simulink model "DPWM_test"  (R2023b)
settings: Solver=VariableStepAuto  StartTime=0.0  StopTime=0.5  MaxStep=0.0001  RelTol=1e-3
libraries: spsMosfetLib x6, spsDCVoltageSourceLib x1, spsGroundLib x1, spsTriangleGeneratorLib x1, spsThreePhaseSeriesRLCBranchLib x1, spsThreePhaseVIMeasurementLib x1, spspowerguiLib x1
settings Model: Creator=oscar  LastModifiedBy=oscar

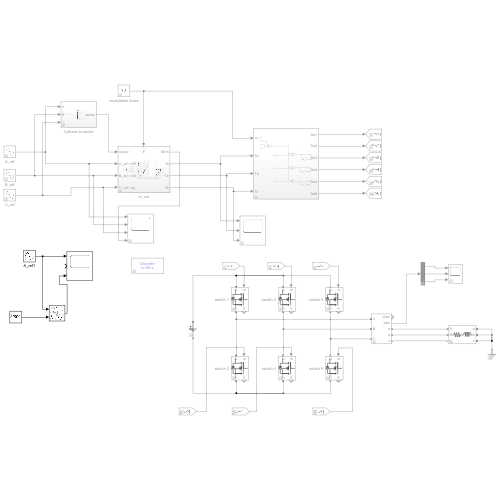
[thumbnail: Simulink's stored preview of the top-level diagram]
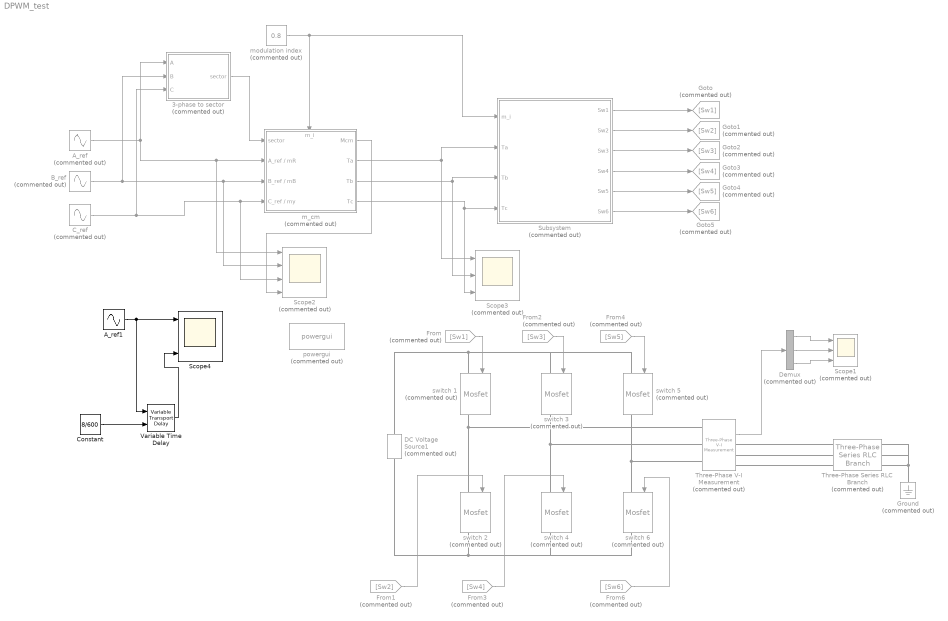
== system DPWM_test ==
  3-phase to sector : Subsystem  Commented=on
  A_ref : Sin  Commented=on  Frequency=2*pi*50  SampleTime=0
  A_ref1 : Sin  Frequency=2*pi*50  SampleTime=0
  B_ref : Sin  Commented=on  Frequency=2*pi*50  Phase=2*pi/3  SampleTime=0
  C_ref : Sin  Commented=on  Frequency=2*pi*50  Phase=4*pi/3  SampleTime=0
  Constant : Constant  Value=8/600
  DC Voltage Source1 : spsDCVoltageSourceLib/DC Voltage Source  Commented=on  Amplitude=100  Measurements=None
  Demux : Demux  Commented=on  Outputs=3
  From : From  Commented=on  GotoTag=Sw1
  From1 : From  Commented=on  GotoTag=Sw2
  From2 : From  Commented=on  GotoTag=Sw3
  From3 : From  Commented=on  GotoTag=Sw4
  From4 : From  Commented=on  GotoTag=Sw5
  From6 : From  Commented=on  GotoTag=Sw6
  Goto : Goto  Commented=on  GotoTag=Sw1
  Goto1 : Goto  Commented=on  GotoTag=Sw2
  Goto2 : Goto  Commented=on  GotoTag=Sw3
  Goto3 : Goto  Commented=on  GotoTag=Sw4
  Goto4 : Goto  Commented=on  GotoTag=Sw5
  Goto5 : Goto  Commented=on  GotoTag=Sw6
  Ground : spsGroundLib/Ground  Commented=on  LConnTagsString=a
  Scope1 : Scope  Commented=on  NumInputPorts=3
  Scope2 : Scope  Commented=on  NumInputPorts=4
  Scope3 : Scope  Commented=on  NumInputPorts=3
  Scope4 : Scope  NumInputPorts=3
  Subsystem : Subsystem  Commented=on
  Three-Phase Series RLC Branch : spsThreePhaseSeriesRLCBranchLib/Three-Phase Series RLC Branch  Commented=on  LConnTagsString=A|B|C  RConnTagsString=A|B|C  BranchType=RL  Resistance=1  Inductance=1e-3  Capacitance=1e-6  Measurements=None
  Three-Phase V-I Measurement : spsThreePhaseVIMeasurementLib/Three-Phase V-I Measurement  Commented=on  VoltageMeasurement=phase-to-ground  SetLabelV=off  LabelV=Vabc  Vpu=off  VpuLL=off  CurrentMeasurement=yes  SetLabelI=off  LabelI=Iabc  Ipu=off  Pbase=100e6  Vbase=500e3  OutputType=Complex  PhasorSimulation=off  PSBequivalent=0
  Variable Time Delay : VariableTransportDelay  VariableDelayType=Variable transport delay  MaximumDelay=10  MaximumPoints=5120
  m_cm : Subsystem  Commented=on
      settings: PortSchema="{\"entries\":[{\"content\":{\"sides\":[{\"content\":{\"connectorIds\":[\"In1\",\"In2\",\"In3\",\"In4\"]},\"type\":\"ConnectorPlacement.EquallySpacedRectSide\",\"uuid\":\"54674ff0-eaad-4175-8630-88aa50651ea8\"},{\"content\":{\"connectorIds\":[\"Out1\",\"Out2\",\"Out3\",\"Out4\"],\"side\":\"RIGHT\"},\"type\":\"ConnectorPlacement.EquallySpacedRectSide\",\"uuid\":\"ebc9f3d9-ae9e-4e4a-bc7f-ec011c2599d1\"},{\"content\":{\"connectorIds\":[\"In5\"],\"side\":\"TOP\"},\"type\":\"ConnectorPlacement.EquallySpacedRectSide\",\"uuid\":\"61633b12-822e-421c-b291-d3bde5d81edf\"}]},\"type\":\"ConnectorPlacement.EquallySpacedConnector\",\"uuid\":\"3ff1106a-c865-4e24-b201-c6220c4a9b86\"}],\"packageUris\":[\"http://schema.mathworks.com/mf0/Connector/R2020b\"],\"version\":\"1.0\"}"
  modulation index : Constant  Commented=on  Value=0.8
  powergui : spspowerguiLib/powergui  Priority=1  Commented=on  SimulationMode=Discrete  SampleTime=1e-6  frequency=60  Iterations=50  frequencyindice=0  Pbase=100e6  ErrMax=1e-4  UnitsV=kV  UnitsW=MW  buscounter=0  FunctionMessages=off  echomessages=off  EnableUseOfTLC=off  CurrentSourceSwitches=off  DisableSnubberDevices=off  DisableRonSwitches=off  DisableVfSwitches=off  DisplayEquations=off  AutomaticDiscreteSolvers=off  SolverType=Tustin/Backward Euler (TBE)  Interpol=off  ExternalGateDelay=off  methode=off  Ts=100  x0status=blocks  SPID=on  SwTol=0  HookPort=off  NonlinearTolerance=1e-4  nMaxIteration=100  ContinueOnMaxIteration=off  RestoreLinks=warning  ResistiveCurrentMeasurement=off  Frange=[0:2:500]  Ylog=off  Xlog=on  ShowGrid=off  save=off  variable=ZData  structure=0  ZoomFFT=off  StartTime=0.0  cycles=1  DisplayStyle=1  fundamental=60  FreqAxis=off  MaxFrequency=1000  frequencyindicesteady=1  RmsSteady=1  display=off
  switch {1..6} (6 alike) : spsMosfetLib/Mosfet  Commented=on  Ron=0.1  Lon=0  Rd=0.01  Vfd=0  IC=0  Rs=1e5  Cs=inf  Measurements=on
  wires:
  From/1 -> switch 1/1
  From1/1 -> switch 2/1
  From2/1 -> switch 3/1
  From3/1 -> switch 4/1
  From4/1 -> switch 5/1
  From6/1 -> switch 6/1
  Subsystem/3(Sw3) -> Goto2/1
  Subsystem/4(Sw4) -> Goto3/1
  Subsystem/5(Sw5) -> Goto4/1
  Demux/1 -> Scope1/1
  Demux/3 -> Scope1/3
  Demux/2 -> Scope1/2
  Three-Phase V-I Measurement/2 -> Demux/1
  A_ref/1 -> 3-phase to sector/1(A), Scope2/1, m_cm/2(A_ref / mR)
  B_ref/1 -> 3-phase to sector/2(B), Scope2/2, m_cm/3(B_ref / mB)
  C_ref/1 -> 3-phase to sector/3(C), Scope2/3, m_cm/4(C_ref / my)
  3-phase to sector/1(sector) -> m_cm/1(sector)
  m_cm/1(Mcm) -> Scope2/4
  m_cm/3(Tb) -> Subsystem/3(Tb), Scope3/2
  m_cm/2(Ta) -> Subsystem/2(Ta), Scope3/1
  m_cm/4(Tc) -> Subsystem/4(Tc), Scope3/3
  Subsystem/1(Sw1) -> Goto/1
  Subsystem/2(Sw2) -> Goto1/1
  Subsystem/6(Sw6) -> Goto5/1
  modulation index/1 -> Subsystem/1(m_i), m_cm/5(m_i)
  A_ref1/1 -> Variable Time Delay/1, Scope4/1
  Variable Time Delay/1 -> Scope4/3
  Constant/1 -> Variable Time Delay/2
  connections:
  DC Voltage Source1/LConn1 -- switch 6/RConn1 -- switch 4/RConn1 -- switch 2/RConn1
  DC Voltage Source1/RConn1 -- switch 1/LConn1 -- switch 3/LConn1 -- switch 5/LConn1
  switch 1/RConn1 -- Three-Phase V-I Measurement/LConn1 -- switch 2/LConn1
  switch 5/RConn1 -- Three-Phase V-I Measurement/LConn3 -- switch 6/LConn1
  switch 3/RConn1 -- Three-Phase V-I Measurement/LConn2 -- switch 4/LConn1
  Three-Phase Series RLC Branch/LConn1 -- Three-Phase V-I Measurement/RConn1
  Three-Phase Series RLC Branch/LConn2 -- Three-Phase V-I Measurement/RConn2
  Three-Phase Series RLC Branch/LConn3 -- Three-Phase V-I Measurement/RConn3
  Ground/LConn1 -- Three-Phase Series RLC Branch/RConn1 -- Three-Phase Series RLC Branch/RConn2 -- Three-Phase Series RLC Branch/RConn3

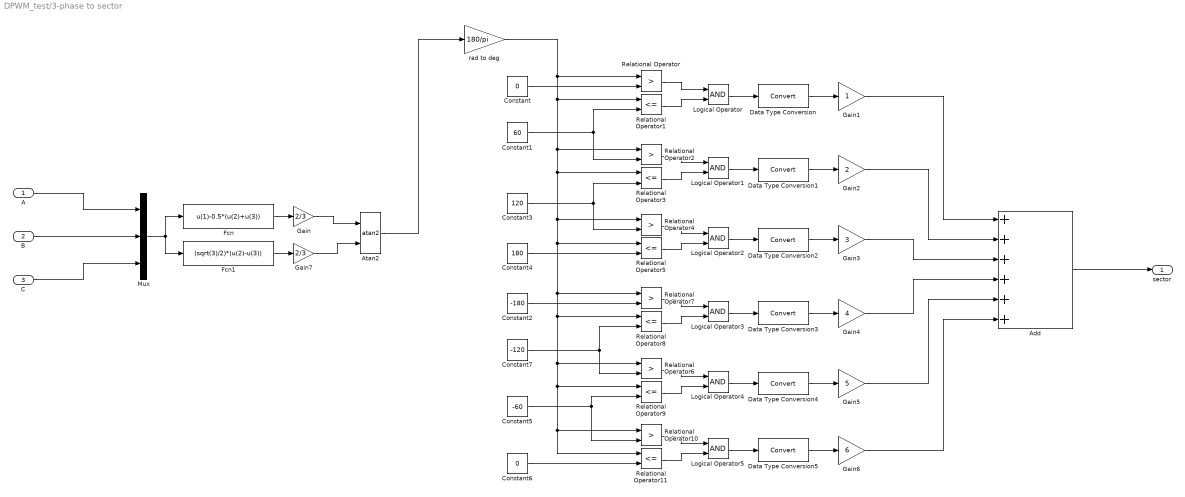
== system DPWM_test/3-phase to sector ==
  A : Inport
  B : Inport  Port=2
  C : Inport  Port=3
  Add : Sum  Inputs=++++++
  Atan2 : Trigonometry  Operator=atan2
  Constant : Constant  Value=0
  Constant1 : Constant  Value=60
  Constant2 : Constant  Value=-180
  Constant3 : Constant  Value=120
  Constant4 : Constant  Value=180
  Constant5 : Constant  Value=-60
  Constant6 : Constant  Value=0
  Constant7 : Constant  Value=-120
  Data Type Conversion{,1..5} (6 alike) : DataTypeConversion  SaturateOnIntegerOverflow=off  RndMeth=Floor
  Fcn : Fcn  Expr=u(1)-0.5*(u(2)+u(3))
  Fcn1 : Fcn  Expr=(sqrt(3)/2)*(u(2)-u(3))
  Gain : Gain  Gain=2/3
  Gain1 : Gain
  Gain2 : Gain  Gain=2
  Gain3 : Gain  Gain=3
  Gain4 : Gain  Gain=4
  Gain5 : Gain  Gain=5
  Gain6 : Gain  Gain=6
  Gain7 : Gain  Gain=2/3
  Logical Operator{,1..5} (6 alike) : Logic  AllPortsSameDT=off  OutDataTypeStr=boolean
  Mux : Mux  Inputs=3
  Relational Operator{,2,4,6..7,10} (6 alike) : RelationalOperator  Operator=>  OutDataTypeStr=boolean  RndMeth=Simplest  InputSameDT=off
  Relational Operator{1,3,5,8..9,11} (6 alike) : RelationalOperator  Operator=<=  OutDataTypeStr=boolean  RndMeth=Simplest  InputSameDT=off
  rad to deg : Gain  Gain=180/pi
  sector : Outport
  wires:
  Relational Operator5/1 -> Logical Operator2/2
  Data Type Conversion5/1 -> Gain6/1
  Data Type Conversion2/1 -> Gain3/1
  Constant/1 -> Relational Operator/2
  Data Type Conversion/1 -> Gain1/1
  Logical Operator3/1 -> Data Type Conversion3/1
  Constant3/1 -> Relational Operator3/2, Relational Operator4/2
  Gain1/1 -> Add/1
  Relational Operator/1 -> Logical Operator/1
  Logical Operator/1 -> Data Type Conversion/1
  Gain6/1 -> Add/6
  Constant2/1 -> Relational Operator7/2
  Logical Operator5/1 -> Data Type Conversion5/1
  Data Type Conversion1/1 -> Gain2/1
  Gain2/1 -> Add/2
  Gain4/1 -> Add/4
  Relational Operator8/1 -> Logical Operator3/2
  Logical Operator2/1 -> Data Type Conversion2/1
  Atan2/1 -> rad to deg/1
  Constant7/1 -> Relational Operator8/2, Relational Operator6/2
  Logical Operator4/1 -> Data Type Conversion4/1
  Relational Operator6/1 -> Logical Operator4/1
  Relational Operator7/1 -> Logical Operator3/1
  Relational Operator2/1 -> Logical Operator1/1
  Constant1/1 -> Relational Operator2/2, Relational Operator1/2
  Data Type Conversion4/1 -> Gain5/1
  Relational Operator4/1 -> Logical Operator2/1
  Relational Operator1/1 -> Logical Operator/2
  Gain3/1 -> Add/3
  rad to deg/1 -> Relational Operator/1, Relational Operator5/1, Relational Operator11/1, Relational Operator10/1, Relational Operator9/1, Relational Operator6/1, Relational Operator8/1, Relational Operator7/1, Relational Operator4/1, Relational Operator3/1, Relational Operator2/1, Relational Operator1/1
  Relational Operator3/1 -> Logical Operator1/2
  Relational Operator11/1 -> Logical Operator5/2
  Constant6/1 -> Relational Operator11/2
  Data Type Conversion3/1 -> Gain4/1
  Constant4/1 -> Relational Operator5/2
  Constant5/1 -> Relational Operator9/2, Relational Operator10/2
  Logical Operator1/1 -> Data Type Conversion1/1
  Add/1 -> sector/1
  Gain5/1 -> Add/5
  Relational Operator10/1 -> Logical Operator5/1
  Relational Operator9/1 -> Logical Operator4/2
  Fcn/1 -> Gain/1
  C/1 -> Mux/3
  Fcn1/1 -> Gain7/1
  B/1 -> Mux/2
  Mux/1 -> Fcn1/1, Fcn/1
  A/1 -> Mux/1
  Gain/1 -> Atan2/1
  Gain7/1 -> Atan2/2

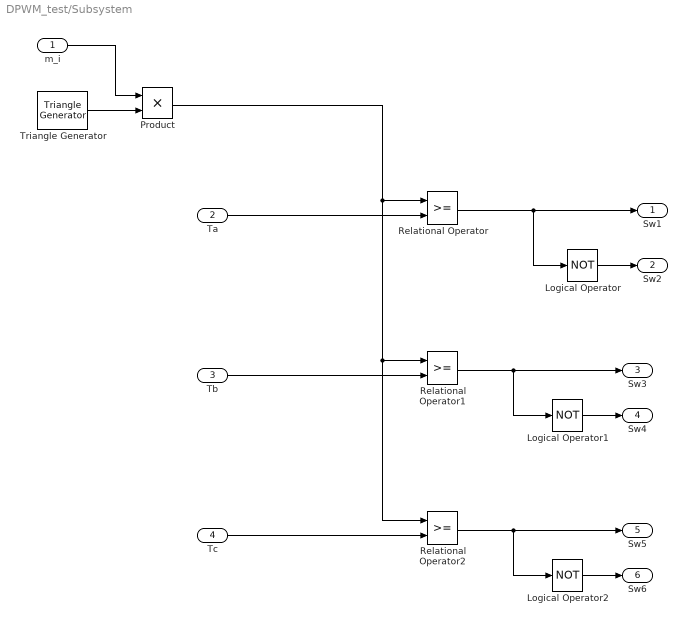
== system DPWM_test/Subsystem ==
  m_i : Inport
  Ta : Inport  Port=2
  Tb : Inport  Port=3
  Tc : Inport  Port=4
  Logical Operator : Logic  Operator=NOT  AllPortsSameDT=off  OutDataTypeStr=boolean
  Logical Operator1 : Logic  Operator=NOT  AllPortsSameDT=off  OutDataTypeStr=boolean
  Logical Operator2 : Logic  Operator=NOT  AllPortsSameDT=off  OutDataTypeStr=boolean
  Product : Product
  Relational Operator : RelationalOperator  OutDataTypeStr=boolean  RndMeth=Simplest  InputSameDT=off
  Relational Operator1 : RelationalOperator  OutDataTypeStr=boolean  RndMeth=Simplest  InputSameDT=off
  Relational Operator2 : RelationalOperator  OutDataTypeStr=boolean  RndMeth=Simplest  InputSameDT=off
  Triangle Generator : spsTriangleGeneratorLib/Triangle Generator  Freq=10e3  Phase=90  Ts=0
  Sw1 : Outport
  Sw2 : Outport  Port=2
  Sw3 : Outport  Port=3
  Sw4 : Outport  Port=4
  Sw5 : Outport  Port=5
  Sw6 : Outport  Port=6
  wires:
  Logical Operator1/1 -> Sw4/1
  Product/1 -> Relational Operator/1, Relational Operator2/1, Relational Operator1/1
  Triangle Generator/1 -> Product/2
  Tb/1 -> Relational Operator1/2
  Relational Operator2/1 -> Sw5/1, Logical Operator2/1
  Logical Operator/1 -> Sw2/1
  Tc/1 -> Relational Operator2/2
  Logical Operator2/1 -> Sw6/1
  Ta/1 -> Relational Operator/2
  Relational Operator1/1 -> Sw3/1, Logical Operator1/1
  Relational Operator/1 -> Sw1/1, Logical Operator/1
  m_i/1 -> Product/1

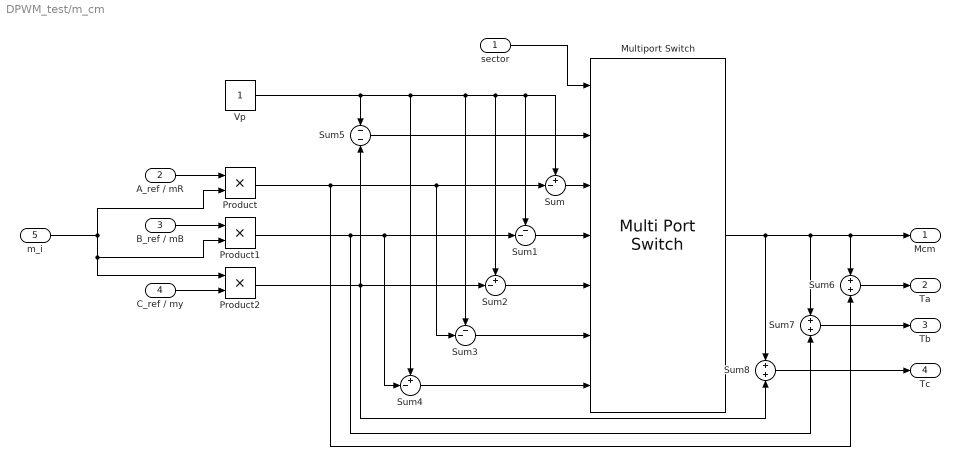
== system DPWM_test/m_cm ==
  sector : Inport
  A_ref / mR : Inport  Port=2
  B_ref / mB : Inport  Port=3
  C_ref / my : Inport  Port=4
  m_i : Inport  Port=5
  Multiport Switch : MultiPortSwitch  Inputs=6  SaturateOnIntegerOverflow=off  InputSameDT=off
  Product : Product
  Product1 : Product
  Product2 : Product
  Sum : Sum  Inputs=+-|
  Sum1 : Sum  Inputs=--|
  Sum2 : Sum  Inputs=+-|
  Sum3 : Sum  Inputs=--|
  Sum4 : Sum  Inputs=+-|
  Sum5 : Sum  Inputs=-|-
  Sum6 : Sum  Inputs=+|+
  Sum7 : Sum  Inputs=+|+
  Sum8 : Sum  Inputs=+|+
  Vp : Constant
  Mcm : Outport
  Ta : Outport  Port=2
  Tb : Outport  Port=3
  Tc : Outport  Port=4
  wires:
  Multiport Switch/1 -> Sum8/1, Sum6/1, Mcm/1, Sum7/1
  sector/1 -> Multiport Switch/1
  Sum/1 -> Multiport Switch/3
  Product/1 -> Sum3/2, Sum/2, Sum6/2
  Sum1/1 -> Multiport Switch/4
  Vp/1 -> Sum5/1, Sum4/1, Sum3/1, Sum2/1, Sum1/1, Sum/1
  Product1/1 -> Sum7/2, Sum4/2, Sum1/2
  Sum2/1 -> Multiport Switch/5
  Product2/1 -> Sum8/2, Sum5/2, Sum2/2
  Sum3/1 -> Multiport Switch/6
  Sum4/1 -> Multiport Switch/7
  Sum5/1 -> Multiport Switch/2
  Sum6/1 -> Ta/1
  Sum7/1 -> Tb/1
  Sum8/1 -> Tc/1
  A_ref / mR/1 -> Product/1
  B_ref / mB/1 -> Product1/1
  C_ref / my/1 -> Product2/2
  m_i/1 -> Product/2, Product2/1, Product1/2
